simulink model "Core_XY_gantry"  (R2022a)
settings: Solver=VariableStepAuto  StartTime=0.0  StopTime=10.0  RelTol=1e-3
undefined symbols (not defined in the file or in its folder): DiscIntNeverNeededParam, Iref, Nstep, Ts
libraries: spsUniversalBridgeLib x4, spsCurrentMeasurementLib x4, spsStepperMotorLib x2
settings Model: Creator=Pc  LastModifiedBy=Pc

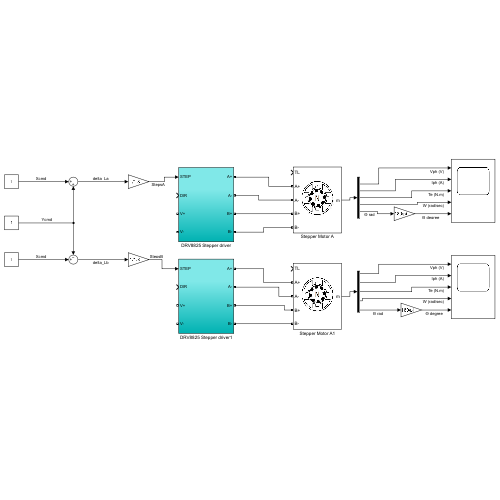
[thumbnail: Simulink's stored preview of the top-level diagram]
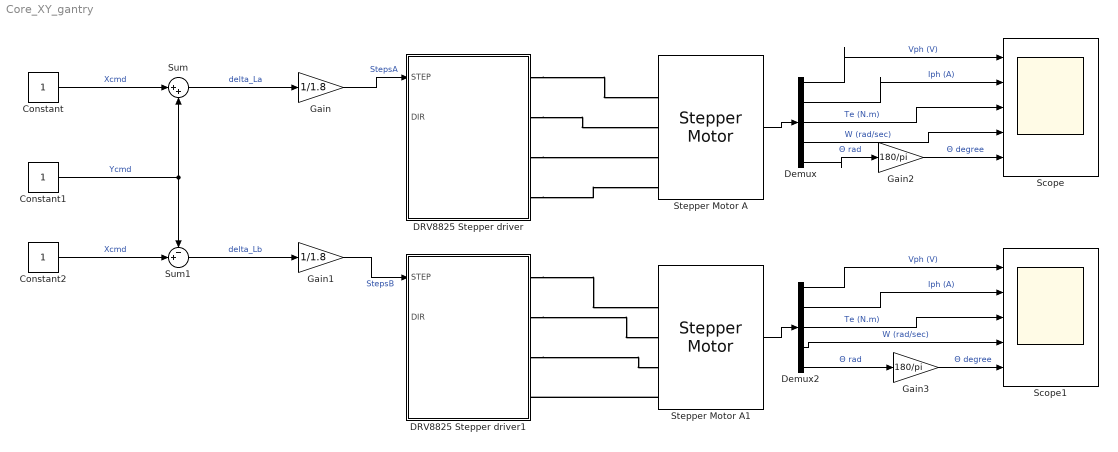
== system Core_XY_gantry ==
  Constant : Constant
  Constant1 : Constant
  Constant2 : Constant
  DRV8825 Stepper driver : Subsystem
  DRV8825 Stepper driver1 : Subsystem
  Demux : Demux  Outputs=5
  Demux2 : Demux  Outputs=5
  Gain : Gain  Gain=1/1.8
  Gain1 : Gain  Gain=1/1.8
  Gain2 : Gain  Gain=180/pi
  Gain3 : Gain  Gain=180/pi
  Scope : Scope  NumInputPorts=5
  Scope1 : Scope  NumInputPorts=5
  Stepper Motor A : spsStepperMotorLib/Stepper Motor  MotorType=Permanent-magnet / Hybrid  NumberOfPhases_1=2  NumberOfPhases_2=3  PresetModel_1=<empty>  PresetModel_2=<empty>  L=10e-3  Lmax=10e-3  Lmin=2e-3  R=1.2  Step_angle=30  Psim=0.04  Tdm=0.02  J=1e-4/5  B=1e-3  w0=0  pos0=0  TsPowergui=0  TsBlock=-1
      settings: SourceProductBaseCode=PS
  Stepper Motor A1 : spsStepperMotorLib/Stepper Motor  MotorType=Permanent-magnet / Hybrid  NumberOfPhases_1=2  NumberOfPhases_2=3  PresetModel_1=<empty>  PresetModel_2=<empty>  L=10e-3  Lmax=10e-3  Lmin=2e-3  R=1.2  Step_angle=30  Psim=0.04  Tdm=0.02  J=1e-4/5  B=1e-3  w0=0  pos0=0  TsPowergui=0  TsBlock=-1
      settings: SourceProductBaseCode=PS
  Sum : Sum  Inputs=|++
  Sum1 : Sum  Inputs=-+|
  wires:
  Constant/1 -> Sum/1  "Xcmd"
  Constant1/1 -> Sum1/1, Sum/2  "Ycmd"
  Constant2/1 -> Sum1/2  "Xcmd"
  Sum/1 -> Gain/1  "delta_La"
  Sum1/1 -> Gain1/1  "delta_Lb"
  Gain1/1 -> DRV8825 Stepper driver1/1(STEP)  "StepsB"
  Gain/1 -> DRV8825 Stepper driver/1(STEP)  "StepsA"
  Stepper Motor A/1 -> Demux/1
  Demux/5 -> Gain2/1  "Θ rad"
  Gain2/1 -> Scope/5  "Θ degree"
  Demux/4 -> Scope/4  "W (rad/sec)"
  Demux/3 -> Scope/3  "Te (N.m)"
  Demux/2 -> Scope/2  "Iph (A)"
  Demux/1 -> Scope/1  "Vph (V)"
  Demux2/2 -> Scope1/2  "Iph (A)"
  Stepper Motor A1/1 -> Demux2/1
  Demux2/5 -> Gain3/1  "Θ rad"
  Demux2/4 -> Scope1/4  "W (rad/sec)"
  Demux2/3 -> Scope1/3  "Te (N.m)"
  Gain3/1 -> Scope1/5  "Θ degree"
  Demux2/1 -> Scope1/1  "Vph (V)"
  connections:
  DRV8825 Stepper driver/RConn1 -- Stepper Motor A/LConn1
  DRV8825 Stepper driver/RConn2 -- Stepper Motor A/LConn2
  DRV8825 Stepper driver/RConn3 -- Stepper Motor A/LConn3
  DRV8825 Stepper driver/RConn4 -- Stepper Motor A/LConn4
  DRV8825 Stepper driver1/RConn1 -- Stepper Motor A1/LConn1
  DRV8825 Stepper driver1/RConn2 -- Stepper Motor A1/LConn2
  DRV8825 Stepper driver1/RConn3 -- Stepper Motor A1/LConn3
  Stepper Motor A1/LConn4 -- DRV8825 Stepper driver1/RConn4

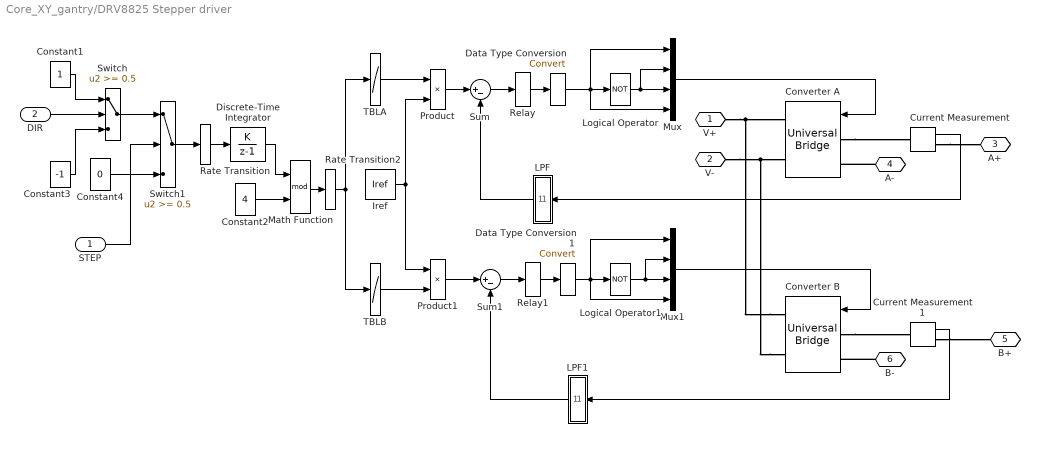
== system Core_XY_gantry/DRV8825 Stepper driver ==
  STEP : Inport
  DIR : Inport  Port=2
  Constant1 : Constant  SampleTime=Ts
  Constant2 : Constant  Value=4  SampleTime=Nstep*Ts
  Constant3 : Constant  Value=-1  SampleTime=Ts
  Constant4 : Constant  Value=0  SampleTime=Ts
  Converter A : spsUniversalBridgeLib/Universal Bridge  Arms=2  SnubberResistance=10000  SnubberCapacitance=inf  Device=MOSFET / Diodes  Ron=1e-3*10  Lon=0  ForwardVoltages="[  0  0  ]"  ForwardVoltage=0  GTOparameters=[ 10e-6 , 20e-6 ]  IGBTparameters=[ 0.5e-6 , 0.5e-6 ]  Measurements=None  Measurements_2=None  converterType=Rectifier
  Converter B : spsUniversalBridgeLib/Universal Bridge  Arms=2  SnubberResistance=10000  SnubberCapacitance=inf  Device=MOSFET / Diodes  Ron=1e-3*10  Lon=0  ForwardVoltages="[  0  0  ]"  ForwardVoltage=0  GTOparameters=[ 10e-6 , 20e-6 ]  IGBTparameters=[ 0.5e-6 , 0.5e-6 ]  Measurements=None  Measurements_2=None  converterType=Rectifier
  Current Measurement : spsCurrentMeasurementLib/Current Measurement  PhasorSimulation=off  OutputType=Complex  PSBequivalent=0
  Current Measurement1 : spsCurrentMeasurementLib/Current Measurement  PhasorSimulation=off  OutputType=Complex  PSBequivalent=0
  Data Type Conversion : DataTypeConversion  SaturateOnIntegerOverflow=off  RndMeth=Floor
  Data Type Conversion1 : DataTypeConversion  SaturateOnIntegerOverflow=off  RndMeth=Floor
  Discrete-Time Integrator : DiscreteIntegrator  IntegratorMethod=Accumulation: Forward Euler  SampleTime=Nstep*Ts  ICPrevOutput=DiscIntNeverNeededParam  ICPrevScaledInput=DiscIntNeverNeededParam
  Iref : Constant  Value=Iref  SampleTime=Ts
  LPF : Subsystem  mask{fc=10000, Ts=Ts}
      mask prompts: fc "Cut-off frequency (Hz)"; Ts "Sampling time (s)"
      mask init:
      | % fa=tf(1,[1/2/pi/fc 1]);
      | % fn=c2d(fa,Ts);
      | % [NN,DD]=tfdata(fn,'v')
      | 
      | NN = [ 0,0.0609];
      | DD = [1.0000,-0.9391];
  LPF1 : Subsystem  mask{fc=10000, Ts=Ts}
      mask prompts: fc "Cut-off frequency (Hz)"; Ts "Sampling time (s)"
      mask init:
      | % fa=tf(1,[1/2/pi/fc 1]);
      | % fn=c2d(fa,Ts);
      | % [NN,DD]=tfdata(fn,'v')
      | 
      | NN = [ 0,0.0609];
      | DD = [1.0000,-0.9391];
  Logical Operator : Logic  Operator=NOT  AllPortsSameDT=off  OutDataTypeStr=boolean
  Logical Operator1 : Logic  Operator=NOT  AllPortsSameDT=off  OutDataTypeStr=boolean
  Math Function : Math  Operator=mod  SignedPower=on  SampleTime=Nstep*Ts
  Mux : Mux
  Mux1 : Mux
  Product : Product  RndMeth=Zero
  Product1 : Product  RndMeth=Zero
  Rate Transition : RateTransition
  Rate Transition2 : RateTransition
  Relay : Relay  OnSwitchValue=0.01  OffSwitchValue=-0.01
  Relay1 : Relay  OnSwitchValue=0.01  OffSwitchValue=-0.01  OutDataTypeStr=Inherit: Inherit via back propagation
  Sum : Sum  Inputs=|+-  OutDataTypeStr=Inherit: Same as first input
  Sum1 : Sum  Inputs=|+-  OutDataTypeStr=Inherit: Same as first input
  Switch : Switch  Threshold=0.5  ZeroCross=off  SampleTime=Ts  SaturateOnIntegerOverflow=off  InputSameDT=off
  Switch1 : Switch  Threshold=0.5  ZeroCross=off  SampleTime=Ts  SaturateOnIntegerOverflow=off  InputSameDT=off
  TBLA : Lookup_n-D  NumberOfTableDimensions=1  BreakpointsForDimension1=[0:3]  BreakpointsForDimension2=[0 571.55 685.8 800.15 914.4 1028.8 1143.1 1257.4 1371.7 1486 1600.3 1714.6 1828.9 1943.2 2057.5 2171.8 2286.1 2400.5 2514.7 2629.1 2743.3 2857.7 2971.9 3086.3 3200.5 3314.9 3429.2]  Table=[1 0 -1 0]  InternalRulePriority=Speed  RndMeth=Simplest
  TBLB : Lookup_n-D  NumberOfTableDimensions=1  BreakpointsForDimension1=[0:3]  BreakpointsForDimension2=[0 571.55 685.8 800.15 914.4 1028.8 1143.1 1257.4 1371.7 1486 1600.3 1714.6 1828.9 1943.2 2057.5 2171.8 2286.1 2400.5 2514.7 2629.1 2743.3 2857.7 2971.9 3086.3 3200.5 3314.9 3429.2]  Table=[0 1 0 -1]  InternalRulePriority=Speed  RndMeth=Simplest
  V+ : PMIOPort  Side=Left
  V- : PMIOPort  Port=2  Side=Left
  A+ : PMIOPort  Port=3  Side=Right
  A- : PMIOPort  Port=4  Side=Right
  B+ : PMIOPort  Port=5  Side=Right
  B- : PMIOPort  Port=6  Side=Right
  wires:
  Constant4/1 -> Switch1/3
  Switch1/1 -> Rate Transition/1
  Switch/1 -> Switch1/1
  STEP/1 -> Switch1/2
  DIR/1 -> Switch/2
  Rate Transition2/1 -> TBLB/1, TBLA/1
  Math Function/1 -> Rate Transition2/1
  Product1/1 -> Sum1/1
  Product/1 -> Sum/1
  Rate Transition/1 -> Discrete-Time Integrator/1
  Constant3/1 -> Switch/3
  Constant1/1 -> Switch/1
  Discrete-Time Integrator/1 -> Math Function/1
  Constant2/1 -> Math Function/2
  Iref/1 -> Product1/1, Product/2
  TBLB/1 -> Product1/2
  TBLA/1 -> Product/1
  LPF1/1(O) -> Sum1/2
  LPF/1(O) -> Sum/2
  Data Type Conversion1/1 -> Mux1/4, Mux1/1, Logical Operator1/1
  Data Type Conversion/1 -> Logical Operator/1, Mux/4, Mux/1
  Current Measurement1/1 -> LPF1/1(I)
  Sum1/1 -> Relay1/1
  Mux1/1 -> Converter B/1
  Logical Operator1/1 -> Mux1/2, Mux1/3
  Relay1/1 -> Data Type Conversion1/1
  Mux/1 -> Converter A/1
  Logical Operator/1 -> Mux/2, Mux/3
  Relay/1 -> Data Type Conversion/1
  Current Measurement/1 -> LPF/1(I)
  Sum/1 -> Relay/1
  connections:
  Converter B/RConn2 -- Converter A/RConn2 -- V-/RConn1
  Converter B/RConn1 -- Converter A/RConn1 -- V+/RConn1
  Current Measurement1/RConn1 -- B+/RConn1
  Converter B/LConn1 -- Current Measurement1/LConn1
  Current Measurement/RConn1 -- A+/RConn1
  Converter A/LConn1 -- Current Measurement/LConn1
  B-/RConn1 -- Converter B/LConn2
  A-/RConn1 -- Converter A/LConn2

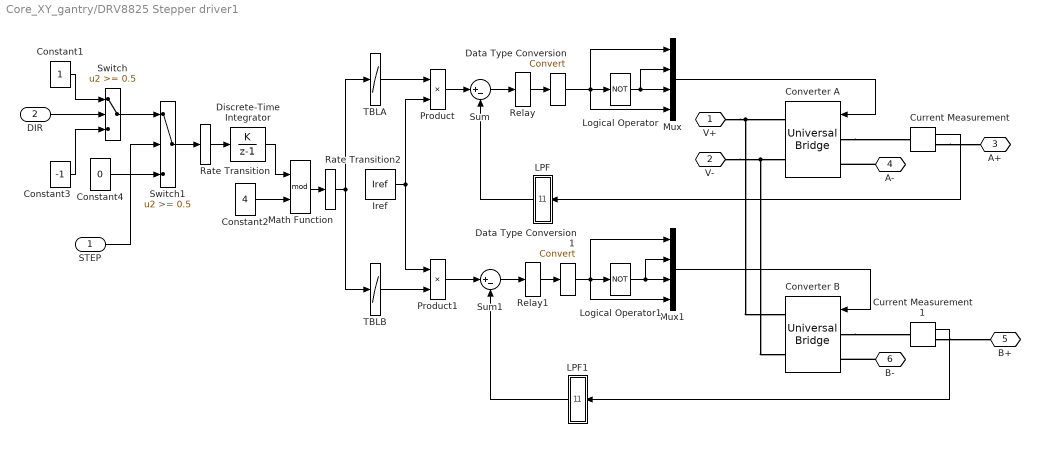
== system Core_XY_gantry/DRV8825 Stepper driver1 ==
  STEP : Inport
  DIR : Inport  Port=2
  Constant1 : Constant  SampleTime=Ts
  Constant2 : Constant  Value=4  SampleTime=Nstep*Ts
  Constant3 : Constant  Value=-1  SampleTime=Ts
  Constant4 : Constant  Value=0  SampleTime=Ts
  Converter A : spsUniversalBridgeLib/Universal Bridge  Arms=2  SnubberResistance=10000  SnubberCapacitance=inf  Device=MOSFET / Diodes  Ron=1e-3*10  Lon=0  ForwardVoltages="[  0  0  ]"  ForwardVoltage=0  GTOparameters=[ 10e-6 , 20e-6 ]  IGBTparameters=[ 0.5e-6 , 0.5e-6 ]  Measurements=None  Measurements_2=None  converterType=Rectifier
  Converter B : spsUniversalBridgeLib/Universal Bridge  Arms=2  SnubberResistance=10000  SnubberCapacitance=inf  Device=MOSFET / Diodes  Ron=1e-3*10  Lon=0  ForwardVoltages="[  0  0  ]"  ForwardVoltage=0  GTOparameters=[ 10e-6 , 20e-6 ]  IGBTparameters=[ 0.5e-6 , 0.5e-6 ]  Measurements=None  Measurements_2=None  converterType=Rectifier
  Current Measurement : spsCurrentMeasurementLib/Current Measurement  PhasorSimulation=off  OutputType=Complex  PSBequivalent=0
  Current Measurement1 : spsCurrentMeasurementLib/Current Measurement  PhasorSimulation=off  OutputType=Complex  PSBequivalent=0
  Data Type Conversion : DataTypeConversion  SaturateOnIntegerOverflow=off  RndMeth=Floor
  Data Type Conversion1 : DataTypeConversion  SaturateOnIntegerOverflow=off  RndMeth=Floor
  Discrete-Time Integrator : DiscreteIntegrator  IntegratorMethod=Accumulation: Forward Euler  SampleTime=Nstep*Ts  ICPrevOutput=DiscIntNeverNeededParam  ICPrevScaledInput=DiscIntNeverNeededParam
  Iref : Constant  Value=Iref  SampleTime=Ts
  LPF : Subsystem  mask{fc=10000, Ts=Ts}
      mask prompts: fc "Cut-off frequency (Hz)"; Ts "Sampling time (s)"
      mask init:
      | % fa=tf(1,[1/2/pi/fc 1]);
      | % fn=c2d(fa,Ts);
      | % [NN,DD]=tfdata(fn,'v')
      | 
      | NN = [ 0,0.0609];
      | DD = [1.0000,-0.9391];
  LPF1 : Subsystem  mask{fc=10000, Ts=Ts}
      mask prompts: fc "Cut-off frequency (Hz)"; Ts "Sampling time (s)"
      mask init:
      | % fa=tf(1,[1/2/pi/fc 1]);
      | % fn=c2d(fa,Ts);
      | % [NN,DD]=tfdata(fn,'v')
      | 
      | NN = [ 0,0.0609];
      | DD = [1.0000,-0.9391];
  Logical Operator : Logic  Operator=NOT  AllPortsSameDT=off  OutDataTypeStr=boolean
  Logical Operator1 : Logic  Operator=NOT  AllPortsSameDT=off  OutDataTypeStr=boolean
  Math Function : Math  Operator=mod  SignedPower=on  SampleTime=Nstep*Ts
  Mux : Mux
  Mux1 : Mux
  Product : Product  RndMeth=Zero
  Product1 : Product  RndMeth=Zero
  Rate Transition : RateTransition
  Rate Transition2 : RateTransition
  Relay : Relay  OnSwitchValue=0.01  OffSwitchValue=-0.01
  Relay1 : Relay  OnSwitchValue=0.01  OffSwitchValue=-0.01  OutDataTypeStr=Inherit: Inherit via back propagation
  Sum : Sum  Inputs=|+-  OutDataTypeStr=Inherit: Same as first input
  Sum1 : Sum  Inputs=|+-  OutDataTypeStr=Inherit: Same as first input
  Switch : Switch  Threshold=0.5  ZeroCross=off  SampleTime=Ts  SaturateOnIntegerOverflow=off  InputSameDT=off
  Switch1 : Switch  Threshold=0.5  ZeroCross=off  SampleTime=Ts  SaturateOnIntegerOverflow=off  InputSameDT=off
  TBLA : Lookup_n-D  NumberOfTableDimensions=1  BreakpointsForDimension1=[0:3]  BreakpointsForDimension2=[0 571.55 685.8 800.15 914.4 1028.8 1143.1 1257.4 1371.7 1486 1600.3 1714.6 1828.9 1943.2 2057.5 2171.8 2286.1 2400.5 2514.7 2629.1 2743.3 2857.7 2971.9 3086.3 3200.5 3314.9 3429.2]  Table=[1 0 -1 0]  InternalRulePriority=Speed  RndMeth=Simplest
  TBLB : Lookup_n-D  NumberOfTableDimensions=1  BreakpointsForDimension1=[0:3]  BreakpointsForDimension2=[0 571.55 685.8 800.15 914.4 1028.8 1143.1 1257.4 1371.7 1486 1600.3 1714.6 1828.9 1943.2 2057.5 2171.8 2286.1 2400.5 2514.7 2629.1 2743.3 2857.7 2971.9 3086.3 3200.5 3314.9 3429.2]  Table=[0 1 0 -1]  InternalRulePriority=Speed  RndMeth=Simplest
  V+ : PMIOPort  Side=Left
  V- : PMIOPort  Port=2  Side=Left
  A+ : PMIOPort  Port=3  Side=Right
  A- : PMIOPort  Port=4  Side=Right
  B+ : PMIOPort  Port=5  Side=Right
  B- : PMIOPort  Port=6  Side=Right
  wires:
  Sum/1 -> Relay/1
  Current Measurement/1 -> LPF/1(I)
  Relay/1 -> Data Type Conversion/1
  Logical Operator/1 -> Mux/3, Mux/2
  Mux/1 -> Converter A/1
  Relay1/1 -> Data Type Conversion1/1
  Logical Operator1/1 -> Mux1/3, Mux1/2
  Mux1/1 -> Converter B/1
  Sum1/1 -> Relay1/1
  Current Measurement1/1 -> LPF1/1(I)
  Data Type Conversion/1 -> Mux/1, Mux/4, Logical Operator/1
  Data Type Conversion1/1 -> Logical Operator1/1, Mux1/1, Mux1/4
  LPF/1(O) -> Sum/2
  LPF1/1(O) -> Sum1/2
  TBLA/1 -> Product/1
  TBLB/1 -> Product1/2
  Iref/1 -> Product/2, Product1/1
  Constant2/1 -> Math Function/2
  Discrete-Time Integrator/1 -> Math Function/1
  Constant1/1 -> Switch/1
  Constant3/1 -> Switch/3
  Rate Transition/1 -> Discrete-Time Integrator/1
  Product/1 -> Sum/1
  Product1/1 -> Sum1/1
  Math Function/1 -> Rate Transition2/1
  Rate Transition2/1 -> TBLA/1, TBLB/1
  DIR/1 -> Switch/2
  STEP/1 -> Switch1/2
  Switch/1 -> Switch1/1
  Switch1/1 -> Rate Transition/1
  Constant4/1 -> Switch1/3
  connections:
  A-/RConn1 -- Converter A/LConn2
  B-/RConn1 -- Converter B/LConn2
  Converter A/LConn1 -- Current Measurement/LConn1
  Current Measurement/RConn1 -- A+/RConn1
  Converter B/LConn1 -- Current Measurement1/LConn1
  Current Measurement1/RConn1 -- B+/RConn1
  V+/RConn1 -- Converter A/RConn1 -- Converter B/RConn1
  V-/RConn1 -- Converter A/RConn2 -- Converter B/RConn2

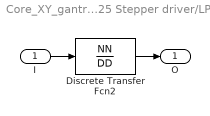
== system Core_XY_gantry/DRV8825 Stepper driver/LPF ==
  I : Inport
  Discrete Transfer Fcn2 : DiscreteTransferFcn  Numerator=NN  Denominator=DD  SampleTime=Ts
  O : Outport  VectorParamsAs1DForOutWhenUnconnected=off
  wires:
  Discrete Transfer Fcn2/1 -> O/1
  I/1 -> Discrete Transfer Fcn2/1

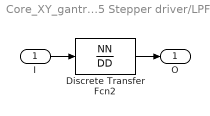
== system Core_XY_gantry/DRV8825 Stepper driver/LPF1 ==
  I : Inport
  Discrete Transfer Fcn2 : DiscreteTransferFcn  Numerator=NN  Denominator=DD  SampleTime=Ts
  O : Outport  VectorParamsAs1DForOutWhenUnconnected=off
  wires:
  I/1 -> Discrete Transfer Fcn2/1
  Discrete Transfer Fcn2/1 -> O/1

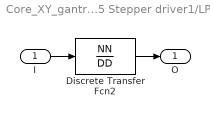
== system Core_XY_gantry/DRV8825 Stepper driver1/LPF ==
  I : Inport
  Discrete Transfer Fcn2 : DiscreteTransferFcn  Numerator=NN  Denominator=DD  SampleTime=Ts
  O : Outport  VectorParamsAs1DForOutWhenUnconnected=off
  wires:
  I/1 -> Discrete Transfer Fcn2/1
  Discrete Transfer Fcn2/1 -> O/1

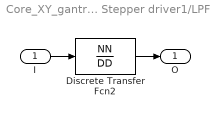
== system Core_XY_gantry/DRV8825 Stepper driver1/LPF1 ==
  I : Inport
  Discrete Transfer Fcn2 : DiscreteTransferFcn  Numerator=NN  Denominator=DD  SampleTime=Ts
  O : Outport  VectorParamsAs1DForOutWhenUnconnected=off
  wires:
  Discrete Transfer Fcn2/1 -> O/1
  I/1 -> Discrete Transfer Fcn2/1
